simulink model "boost_impedance_scan"  (R2024b)
settings: Solver=FixedStepAuto  StartTime=0.0  StopTime=3.25  FixedStep=2.5e-5  MaxStep=5e-7  RelTol=1e-3
values from neighbouring files (symbols this model uses):
  Cf = (Iload0 * (1-D0))/(fs * 0.8)    (= 0.00012109375)    [boost_control_design.m]
  D0 = Vin0/Vdc0    (= 0.5)    [boost_control_design.m]
  fsamp = 20e3    (= 20000)    [boost_control_design.m]
  Iload0 = P0/Vdc0    (= 3.875)    [boost_control_design.m]
  Imax = 2*iLf0    (= 15.5)    [boost_control_design.m]
  kpi = wBWi*Lf    (= 4.86440152814)    [boost_control_design.m]
  kpu = wBWu*Cdc/D0    (= 0.819327364056)    [boost_control_design.m]
  Lf = 1/fs*1/(0.4*iLf0)*(1-0.5)*Vdc0    (= 0.000387096774194)    [boost_control_design.m]
  rCdc = 0.02    [boost_control_design.m]
  Uout0 = Vin0    (= 24)    [boost_control_design.m]
  Vdc0 = 48    [boost_control_design.m]
undefined symbols (not defined in the file or in its folder): DenAD, DenLP, kad, kd, NumAD, NumLP, Ts
libraries: simulink x4, spsSeriesRLCBranchLib x3, spsCurrentMeasurementLib x2, spsIGBTDiodeLib x2, spsControlledCurrentSourceLib x1, spsDCVoltageSourceLib x1, spsVoltageMeasurementLib x1, sps_lib x1
settings Model: Creator=CHMASCH32  LastModifiedBy=anshg
settings OptimizationCC: ReuseModelBlockBuffer=off
settings RTWCC: GPUComputeCapability=3.5

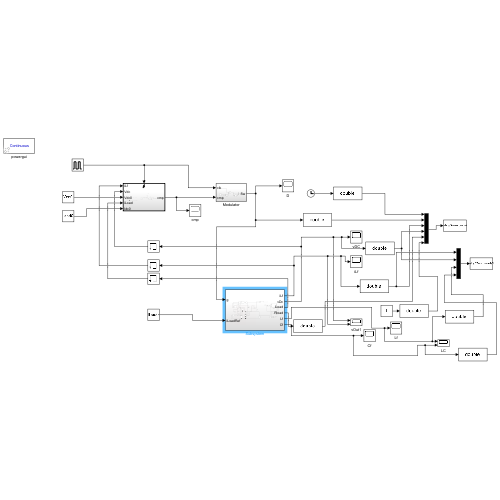
[thumbnail: Simulink's stored preview of the top-level diagram]
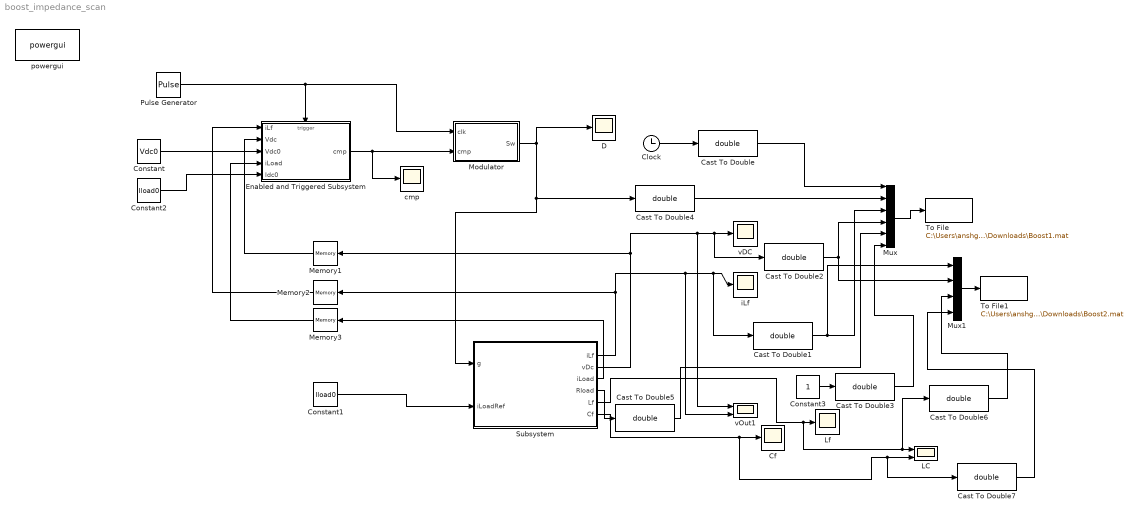
== system boost_impedance_scan ==
  Cast To Double{,1..7} (8 alike) : DataTypeConversion  OutDataTypeStr=double  SaturateOnIntegerOverflow=off  RndMeth=Floor
  Cf : Scope
  Clock : Clock
  Constant : Constant  Value=Vdc0
  Constant1 : Constant  Value=Iload0
  Constant2 : Constant  Value=Iload0
  Constant3 : Constant
  D : Scope
  Enabled and Triggered Subsystem : Subsystem  TreatAsAtomicUnit=on
  LC : Scope  NumInputPorts=2
  Lf : Scope
  Memory1 : Memory
  Memory2 : Memory
  Memory3 : Memory
  Modulator : Subsystem
  Mux : Mux  Inputs=6
  Mux1 : Mux
  Pulse Generator : DiscretePulseGenerator  PulseType=Time based  Period=1/fsamp  PulseWidth=50
  Subsystem : Subsystem
  To File : ToFile  Filename=C:\Users\anshg\Downloads\Boost1.mat  MatrixName=ans1
  To File1 : ToFile  Filename=C:\Users\anshg\Downloads\Boost2.mat  MatrixName=ans1
  cmp : Scope
  iLf : Scope
  powergui : sps_lib/powergui  Priority=1  SimulationMode=Continuous  SampleTime=50e-6  frequency=60  Iterations=50  frequencyindice=0  Pbase=100e6  ErrMax=1e-4  UnitsV=kV  UnitsW=MW  buscounter=0  FunctionMessages=off  echomessages=off  EnableUseOfTLC=off  CurrentSourceSwitches=off  DisableSnubberDevices=off  DisableRonSwitches=off  DisableVfSwitches=off  DisplayEquations=off  AutomaticDiscreteSolvers=off  SolverType=Tustin/Backward Euler (TBE)  Interpol=off  ExternalGateDelay=off  methode=off  Ts=100  x0status=blocks  SPID=on  SwTol=0  HookPort=off  NonlinearTolerance=1e-4  nMaxIteration=100  ContinueOnMaxIteration=off  RestoreLinks=warning  ResistiveCurrentMeasurement=off  Frange=[0:2:500]  Ylog=off  Xlog=on  ShowGrid=off  save=off  variable=ZData  structure=0  ZoomFFT=off  StartTime=0.0  cycles=1  DisplayStyle=1  fundamental=60  FreqAxis=off  MaxFrequency=1000  frequencyindicesteady=1  RmsSteady=1  display=off
  vDC : Scope
  vOut1 : Scope  NumInputPorts=2
  wires:
  Pulse Generator/1 -> Enabled and Triggered Subsystem/Trigger, Modulator/1(clk)
  Enabled and Triggered Subsystem/1(cmp) -> cmp/1, Modulator/2(cmp)
  Modulator/1(Sw) -> Cast To Double4/1, Subsystem/1(g), D/1
  Subsystem/1(iLf) -> vOut1/2, Cast To Double1/1, iLf/1, Memory2/1
  Subsystem/2(vDc) -> vOut1/1, Cast To Double2/1, vDC/1, Memory1/1
  Constant/1 -> Enabled and Triggered Subsystem/3(Vdc0)
  Memory1/1 -> Enabled and Triggered Subsystem/2(Vdc)
  Memory2/1 -> Enabled and Triggered Subsystem/1(iLf)
  Subsystem/3(iLoad) -> Memory3/1
  Memory3/1 -> Enabled and Triggered Subsystem/4(iLoad)
  Constant2/1 -> Enabled and Triggered Subsystem/5(Idc0)
  Constant1/1 -> Subsystem/2(iLoadRef)
  Clock/1 -> Cast To Double/1
  Cast To Double/1 -> Mux/1
  Cast To Double4/1 -> Mux/2
  Cast To Double1/1 -> Mux1/1, Mux/3
  Cast To Double2/1 -> Mux/4, Mux1/2
  Constant3/1 -> Cast To Double3/1
  Cast To Double3/1 -> Mux/6
  Subsystem/4(Rload) -> Cast To Double5/1
  Cast To Double5/1 -> Mux/5
  Mux/1 -> To File/1
  Subsystem/5(Lf) -> Cast To Double6/1, LC/1, Lf/1
  Subsystem/6(Cf) -> Cast To Double7/1, LC/2, Cf/1
  Mux1/1 -> To File1/1
  Cast To Double6/1 -> Mux1/3
  Cast To Double7/1 -> Mux1/4

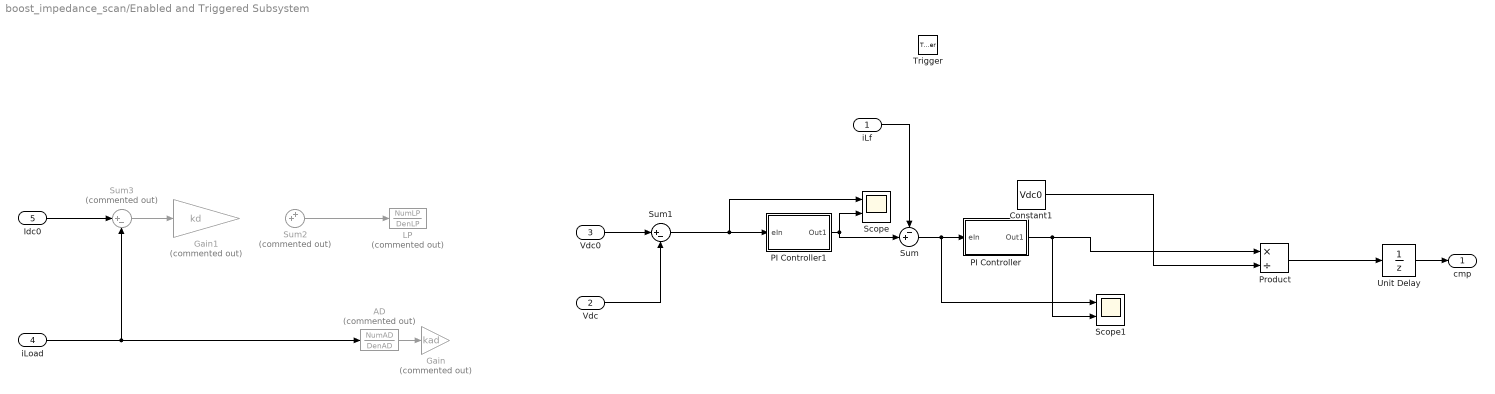
== system boost_impedance_scan/Enabled and Triggered Subsystem ==
  iLf : Inport
  Vdc : Inport  Port=2
  Vdc0 : Inport  Port=3
  iLoad : Inport  Port=4
  Idc0 : Inport  Port=5
  Trigger : TriggerPort  VariantControl=(inherit)
  AD : DiscreteTransferFcn  Commented=on  Numerator=NumAD  Denominator=DenAD
  Constant1 : Constant  Value=Vdc0
  Gain : Gain  Commented=on  Gain=kad
  Gain1 : Gain  Commented=on  Gain=kd
  LP : DiscreteTransferFcn  Commented=on  Numerator=NumLP  Denominator=DenLP
  PI Controller : Subsystem
  PI Controller1 : Subsystem
  Product : Product  Inputs=*/
  Scope : Scope  NumInputPorts=2
  Scope1 : Scope  NumInputPorts=2
  Sum : Sum  Inputs=-+|
  Sum1 : Sum  Inputs=|+-
  Sum2 : Sum  Commented=on  Inputs=++|
  Sum3 : Sum  Commented=on  Inputs=|+-
  Unit Delay : UnitDelay  InitialCondition=D0  SampleTime=-1  HasFrameUpgradeWarning=on
  cmp : Outport
  wires:
  Unit Delay/1 -> cmp/1
  Sum/1 -> Scope1/1, PI Controller/1(eIn)
  iLf/1 -> Sum/1
  Vdc/1 -> Sum1/2
  Sum1/1 -> Scope/1, PI Controller1/1(eIn)
  PI Controller/1(Out1) -> Scope1/2, Product/1
  Product/1 -> Unit Delay/1
  Constant1/1 -> Product/2
  AD/1 -> Gain/1
  iLoad/1 -> Sum3/2, AD/1
  PI Controller1/1(Out1) -> Scope/2, Sum/2
  Sum2/1 -> LP/1
  Sum3/1 -> Gain1/1
  Idc0/1 -> Sum3/1
  Vdc0/1 -> Sum1/1

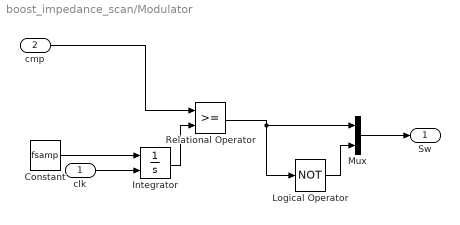
== system boost_impedance_scan/Modulator ==
  clk : Inport
  cmp : Inport  Port=2
  Constant : Constant  Value=fsamp
  Integrator : Integrator  ExternalReset=rising
  Logical Operator : Logic  Operator=NOT  AllPortsSameDT=off  OutDataTypeStr=boolean
  Mux : Mux  Inputs=2
  Relational Operator : RelationalOperator  OutDataTypeStr=boolean  RndMeth=Simplest  InputSameDT=off
  Sw : Outport
  wires:
  Constant/1 -> Integrator/1
  Integrator/1 -> Relational Operator/2
  Relational Operator/1 -> Mux/1, Logical Operator/1
  clk/1 -> Integrator/2
  cmp/1 -> Relational Operator/1
  Mux/1 -> Sw/1
  Logical Operator/1 -> Mux/2

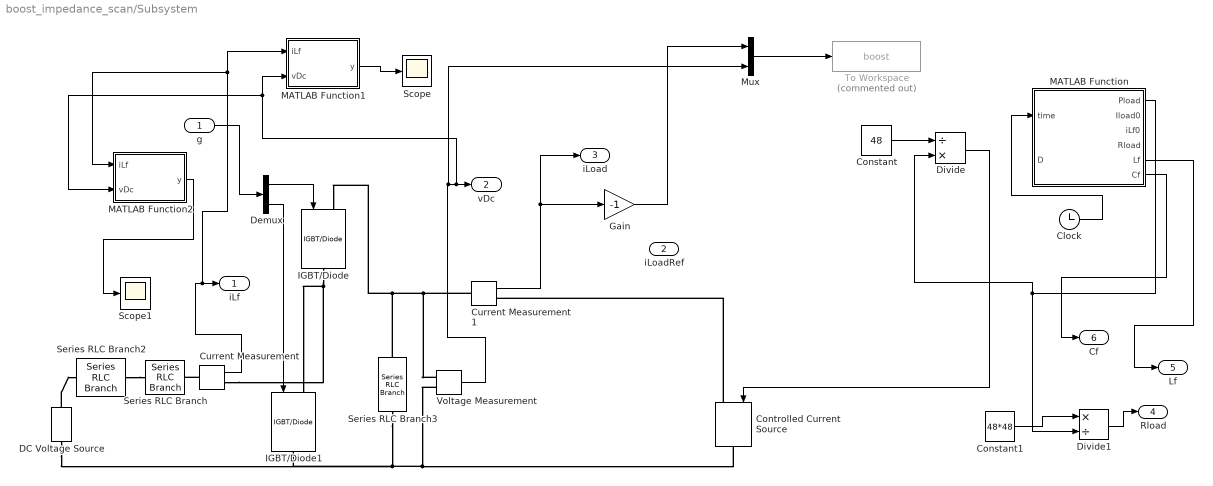
== system boost_impedance_scan/Subsystem ==
  g : Inport
  iLoadRef : Inport  Port=2
  Clock : Clock
  Constant : Constant  Value=48
  Constant1 : Constant  Value=48*48
  Controlled Current Source : spsControlledCurrentSourceLib/Controlled Current Source  Initialize=on  Source_Type=AC  Amplitude=0  Phase=0  Frequency=0  Measurements=None
  Current Measurement : spsCurrentMeasurementLib/Current Measurement  PhasorSimulation=off  OutputType=Complex  PSBequivalent=0
  Current Measurement1 : spsCurrentMeasurementLib/Current Measurement  PhasorSimulation=off  OutputType=Complex  PSBequivalent=0
  DC Voltage Source : spsDCVoltageSourceLib/DC Voltage Source  Amplitude=Uout0  Measurements=None
  Demux : Demux  Outputs=2
  Divide : Product  Inputs=/*
  Divide1 : Product  Inputs=*/
  Gain : Gain  Gain=-1
  IGBT/Diode : spsIGBTDiodeLib/IGBT//Diode  Ron=1e-3  Rs=1e5  Cs=inf  Measurements=off
  IGBT/Diode1 : spsIGBTDiodeLib/IGBT//Diode  Ron=0.221  Rs=1e5  Cs=inf  Measurements=off
  MATLAB Function : MATLAB Function  TreatAsAtomicUnit=on
  MATLAB Function1 : MATLAB Function  TreatAsAtomicUnit=on
  MATLAB Function2 : MATLAB Function  TreatAsAtomicUnit=on
  Mux : Mux  Inputs=2
  Scope : Scope
  Scope1 : Scope
  Series RLC Branch : spsSeriesRLCBranchLib/Series RLC Branch  LConnTagsString=__new0  RConnTagsString=__new0  BranchType=L  Resistance=1  Inductance=Lf  SetiL0=on  InitialCurrent=iLf0  Capacitance=1e-6  Setx0=off  InitialVoltage=0  Measurements=None
  Series RLC Branch2 : spsSeriesRLCBranchLib/Series RLC Branch  LConnTagsString=__new0  RConnTagsString=__new0  BranchType=R  Resistance=0.314  Inductance=1e-3  SetiL0=off  InitialCurrent=0  Capacitance=1e-6  Setx0=off  InitialVoltage=0  Measurements=None
  Series RLC Branch3 : spsSeriesRLCBranchLib/Series RLC Branch  LConnTagsString=__new0  RConnTagsString=__new0  BranchType=RC  Resistance=rCdc  Inductance=1e-3  SetiL0=off  InitialCurrent=0  Capacitance=Cf  Setx0=on  InitialVoltage=Vdc0  Measurements=None
  To Workspace : ToWorkspace  Commented=on  VariableName=boost  SaveFormat=Timeseries  SampleTime=Ts
  Voltage Measurement : spsVoltageMeasurementLib/Voltage Measurement  PhasorSimulation=off  OutputType=Complex  PSBequivalent=0
  iLf : Outport
  vDc : Outport  Port=2
  iLoad : Outport  Port=3
  Rload : Outport  Port=4
  Lf : Outport  Port=5
  Cf : Outport  Port=6
  wires:
  Current Measurement/1 -> MATLAB Function2/1(iLf), MATLAB Function1/1(iLf), iLf/1
  Current Measurement1/1 -> Gain/1, iLoad/1
  g/1 -> Demux/1
  Demux/1 -> IGBT/Diode/1
  Demux/2 -> IGBT/Diode1/1
  Mux/1 -> To Workspace/1
  Gain/1 -> Mux/1
  Voltage Measurement/1 -> Mux/2, MATLAB Function2/2(vDc), MATLAB Function1/2(vDc), vDc/1
  Constant/1 -> Divide/1
  Clock/1 -> MATLAB Function/1(time)
  MATLAB Function/1(Pload) -> Divide/2, Divide1/2
  Divide/1 -> Controlled Current Source/1
  Constant1/1 -> Divide1/1
  Divide1/1 -> Rload/1
  MATLAB Function/5(Lf) -> Lf/1
  MATLAB Function/6(Cf) -> Cf/1
  MATLAB Function1/1(y) -> Scope/1
  MATLAB Function2/1(y) -> Scope1/1
  connections:
  IGBT/Diode/RConn1 -- Current Measurement/RConn1 -- IGBT/Diode1/LConn1
  Voltage Measurement/LConn2 -- DC Voltage Source/LConn1 -- IGBT/Diode1/RConn1 -- Series RLC Branch3/RConn1 -- Controlled Current Source/RConn1
  Voltage Measurement/LConn1 -- Current Measurement1/LConn1 -- IGBT/Diode/LConn1 -- Series RLC Branch3/LConn1
  Current Measurement/LConn1 -- Series RLC Branch/RConn1
  Controlled Current Source/LConn1 -- Current Measurement1/RConn1
  Series RLC Branch2/RConn1 -- Series RLC Branch/LConn1
  DC Voltage Source/RConn1 -- Series RLC Branch2/LConn1

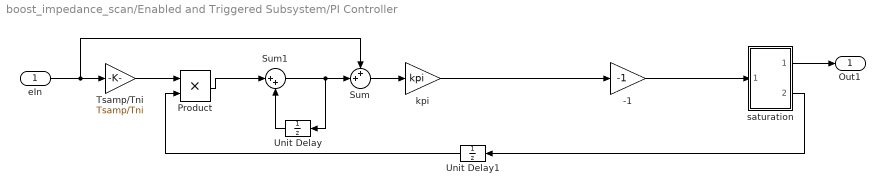
== system boost_impedance_scan/Enabled and Triggered Subsystem/PI Controller ==
  eIn : Inport
  -1 : Gain  Gain=-1
  Product : Product  OutDataTypeStr=double  RndMeth=Zero
  Sum : Sum  Inputs=++|
  Sum1 : Sum  Inputs=|++
  Tsamp/Tni : Gain  Gain=Tsamp/Tni  OutDataTypeStr=double
  Unit Delay : UnitDelay  SampleTime=-1  HasFrameUpgradeWarning=on
  Unit Delay1 : UnitDelay  SampleTime=-1  HasFrameUpgradeWarning=on
  kpi : Gain  Gain=kpi
  saturation : Subsystem
  Out1 : Outport  VectorParamsAs1DForOutWhenUnconnected=off
  wires:
  Sum/1 -> kpi/1
  Tsamp/Tni/1 -> Product/1
  saturation/1(sig_sat) -> Out1/1
  kpi/1 -> -1/1
  Sum1/1 -> Sum/2, Unit Delay/1
  Unit Delay/1 -> Sum1/2
  Product/1 -> Sum1/1
  saturation/2(!sat) -> Unit Delay1/1
  Unit Delay1/1 -> Product/2
  eIn/1 -> Tsamp/Tni/1, Sum/1
  -1/1 -> saturation/1(sig_in)

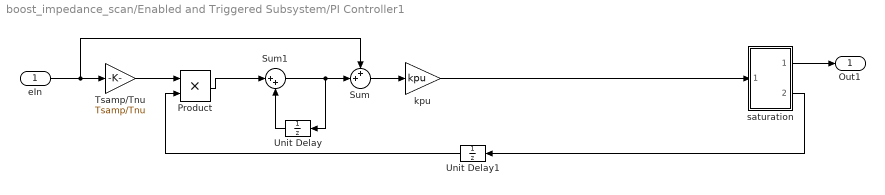
== system boost_impedance_scan/Enabled and Triggered Subsystem/PI Controller1 ==
  eIn : Inport
  Product : Product  OutDataTypeStr=double  RndMeth=Zero
  Sum : Sum  Inputs=++|
  Sum1 : Sum  Inputs=|++
  Tsamp/Tnu : Gain  Gain=Tsamp/Tnu  OutDataTypeStr=double
  Unit Delay : UnitDelay  SampleTime=-1  HasFrameUpgradeWarning=on
  Unit Delay1 : UnitDelay  SampleTime=-1  HasFrameUpgradeWarning=on
  kpu : Gain  Gain=kpu
  saturation : Subsystem
  Out1 : Outport  VectorParamsAs1DForOutWhenUnconnected=off
  wires:
  eIn/1 -> Sum/1, Tsamp/Tnu/1
  Unit Delay1/1 -> Product/2
  saturation/2(!sat) -> Unit Delay1/1
  Product/1 -> Sum1/1
  Unit Delay/1 -> Sum1/2
  Sum1/1 -> Unit Delay/1, Sum/2
  saturation/1(sig_sat) -> Out1/1
  Tsamp/Tnu/1 -> Product/1
  Sum/1 -> kpu/1
  kpu/1 -> saturation/1(sig_in)

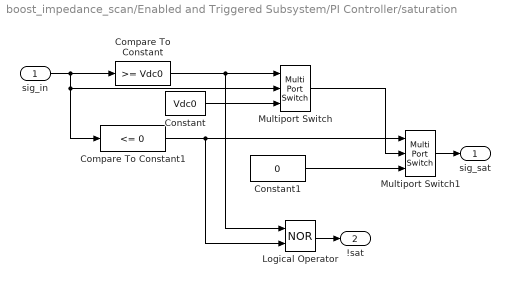
== system boost_impedance_scan/Enabled and Triggered Subsystem/PI Controller/saturation ==
  sig_in : Inport
  Compare To Constant : simulink/Logic and Bit Operations/Compare To Constant  relop=>=  const=Vdc0  OutDataTypeStr=boolean  ZeroCross=off
  Compare To Constant1 : simulink/Logic and Bit Operations/Compare To Constant  relop=<=  const=0  OutDataTypeStr=boolean  ZeroCross=off
  Constant : Constant  Value=Vdc0
  Constant1 : Constant  Value=0
  Logical Operator : Logic  Operator=NOR  AllPortsSameDT=off  OutDataTypeStr=boolean
  Multiport Switch : MultiPortSwitch  DataPortOrder=Zero-based contiguous  Inputs=2  zeroidx=on  SaturateOnIntegerOverflow=off  InputSameDT=off
  Multiport Switch1 : MultiPortSwitch  DataPortOrder=Zero-based contiguous  Inputs=2  zeroidx=on  SaturateOnIntegerOverflow=off  InputSameDT=off
  sig_sat : Outport  VectorParamsAs1DForOutWhenUnconnected=off
  !sat : Outport  Port=2  VectorParamsAs1DForOutWhenUnconnected=off
  wires:
  Compare To Constant/1 -> Multiport Switch/1, Logical Operator/1
  sig_in/1 -> Compare To Constant/1, Multiport Switch/2, Compare To Constant1/1
  Compare To Constant1/1 -> Multiport Switch1/1, Logical Operator/2
  Multiport Switch/1 -> Multiport Switch1/2
  Constant1/1 -> Multiport Switch1/3
  Constant/1 -> Multiport Switch/3
  Multiport Switch1/1 -> sig_sat/1
  Logical Operator/1 -> !sat/1

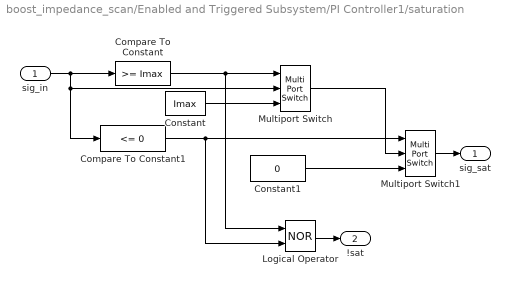
== system boost_impedance_scan/Enabled and Triggered Subsystem/PI Controller1/saturation ==
  sig_in : Inport
  Compare To Constant : simulink/Logic and Bit Operations/Compare To Constant  relop=>=  const=Imax  OutDataTypeStr=boolean  ZeroCross=off
  Compare To Constant1 : simulink/Logic and Bit Operations/Compare To Constant  relop=<=  const=0  OutDataTypeStr=boolean  ZeroCross=off
  Constant : Constant  Value=Imax
  Constant1 : Constant  Value=0
  Logical Operator : Logic  Operator=NOR  AllPortsSameDT=off  OutDataTypeStr=boolean
  Multiport Switch : MultiPortSwitch  DataPortOrder=Zero-based contiguous  Inputs=2  zeroidx=on  SaturateOnIntegerOverflow=off  InputSameDT=off
  Multiport Switch1 : MultiPortSwitch  DataPortOrder=Zero-based contiguous  Inputs=2  zeroidx=on  SaturateOnIntegerOverflow=off  InputSameDT=off
  sig_sat : Outport  VectorParamsAs1DForOutWhenUnconnected=off
  !sat : Outport  Port=2  VectorParamsAs1DForOutWhenUnconnected=off
  wires:
  Logical Operator/1 -> !sat/1
  Multiport Switch1/1 -> sig_sat/1
  Constant/1 -> Multiport Switch/3
  Constant1/1 -> Multiport Switch1/3
  Multiport Switch/1 -> Multiport Switch1/2
  Compare To Constant1/1 -> Logical Operator/2, Multiport Switch1/1
  sig_in/1 -> Compare To Constant1/1, Multiport Switch/2, Compare To Constant/1
  Compare To Constant/1 -> Logical Operator/1, Multiport Switch/1

== matlab function boost_impedance_scan/Subsystem/MATLAB Function1 ==
  data: iLf input; y output; vDc input
function y = predictOutput(iLf, vDc)
    
    coder.extrinsic('pyrun');
    
    persistent model;
    
    y = 0.0;
    
    if isempty(model)
        % Use pyrun to load the model with weights_only=False
        pyrun('import torch; model = torch.load("C:/Users/anshg/Downloads/ml models/ Lmodel.pth", weights_only=False)');
        model = pyrun('model', 'model'); 
    end
    
    pyrun('import numpy; np_array = numpy.array([[float(iLf), float(vDc), 0.0, 0.0, 0.0, 0.0, 0.0, 0.0, 0.0]], dtype=numpy.float32)', 'iLf', iLf, 'vDc', vDc);
    inputData = pyrun('np_array', 'np_array'); % Retrieve the NumPy array
    
    prediction = pyrun('prediction = model.predict(np_array)', 'prediction', 'model', model, 'np_array', inputData);
    
    y = double(prediction);
end

== matlab function boost_impedance_scan/Subsystem/MATLAB Function ==
  data: time input; Pload output; Iload0 output; iLf0 output; D input; Rload output; Lf output; Cf output
function [Pload, Iload0, iLf0, Rload, Lf, Cf] = updateParameters(time, D)
    % Define the base sampling time (seconds)
    Ts = 2.5e-5;     
    % Number of samples for each Pload value
    samples_per_P = 1000;
    
    % Generate Pload values from 70 to 200 (inclusive)
    Pload_values = 10:1:170;
    
    % Calculate the time interval for each Pload value
    interval = samples_per_P * Ts;  % 1000 samples per Pload
    
    % Generate corresponding time points for the ramp changes
    % Each Pload holds for 'interval' seconds
    time_points = 0 : interval : interval*(length(Pload_values)-1);
    
    % Default Pload value is the last one (if time exceeds all defined points)
    Pload = Pload_values(end);
    
    % Determine the appropriate Pload based on current time
    for i = 1:length(time_points)-1
        if time < time_points(i+1)
            Pload = Pload_values(i);
            break;
        end
    end
    
    % Recalculate dependent parameters
    Uout0 = 48;                    % Constant output voltage
    Iload0 = Pload / Uout0;         % Load current based on Pload
    iLf0 = Iload0 / (1 - D);        % Inductor current (steady state assumption)
    Rload = (Uout0^2) / Pload;       % Derived load resistance
    fs = 20000;                    % Switching frequency
    Lf = (1 / fs) * (1 / (0.4 * iLf0)) * (1 - 0.5) * Uout0;
    Cf = (Iload0 * (1 - D)) / (fs * 0.8);
end

== matlab function boost_impedance_scan/Subsystem/MATLAB Function2 ==
  data: iLf input; y output; vDc input
function y = predictOutput(iLf, vDc)
    
    coder.extrinsic('pyrun');
    
    persistent model;
    
    y = 0.0;
    
    if isempty(model)
        % Use pyrun to load the model with weights_only=False
        pyrun('import torch; model = torch.load("C:/Users/anshg/Downloads/ml models/ Cmodel.pth", weights_only=False)');
        model = pyrun('model', 'model'); 
    end
    
    pyrun('import numpy; np_array = numpy.array([[float(iLf), float(vDc), 0.0, 0.0, 0.0, 0.0, 0.0, 0.0, 0.0]], dtype=numpy.float32)', 'iLf', iLf, 'vDc', vDc);
    inputData = pyrun('np_array', 'np_array'); % Retrieve the NumPy array
    
    prediction = pyrun('prediction = model.predict(np_array)', 'prediction', 'model', model, 'np_array', inputData);
    
    y = double(prediction);
end
